simulink model "assignment_4"  (R2020b)
settings: Solver=VariableStepAuto  StartTime=0.0  StopTime=10.0  RelTol=1e-3
values from neighbouring files (symbols this model uses):
  b = 3.5077E-6    [dict1.sldd]
  J = 3.2284E-6    [dict1.sldd]
  K = 0.0274    [dict1.sldd]
  L = 2.75E-6    [dict1.sldd]
  R = 4.0    [dict1.sldd]
settings Model: Creator=Sudhanshu  LastModifiedBy=Sudhanshu

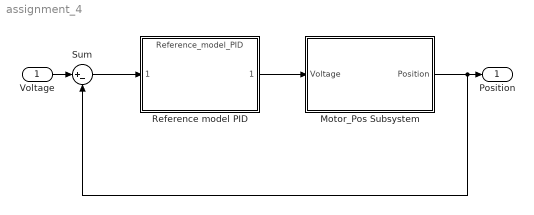
== system assignment_4 ==
  Voltage : Inport
  Motor_Pos Subsystem : Subsystem
  Reference model PID : ModelReference  ModelNameDialog=Reference_model_PID  SimulationMode=Normal  ModelReferenceVersion=1.4
  Sum : Sum  Inputs=|+-
  Position : Outport
  wires:
  Motor_Pos Subsystem/1(Position) -> Sum/2, Position/1
  Voltage/1 -> Sum/1
  Sum/1 -> Reference model PID/1
  Reference model PID/1 -> Motor_Pos Subsystem/1(Voltage)

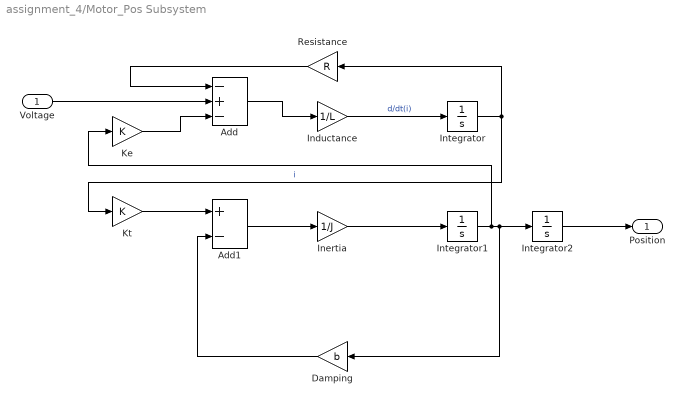
== system assignment_4/Motor_Pos Subsystem ==
  Voltage : Inport
  Add : Sum  Inputs=-+-
  Add1 : Sum  Inputs=+-
  Damping : Gain  Gain=b
  Inductance : Gain  Gain=1/L
  Inertia : Gain  Gain=1/J
  Integrator : Integrator
  Integrator1 : Integrator
  Integrator2 : Integrator
  Ke : Gain  Gain=K
  Kt : Gain  Gain=K
  Resistance : Gain  Gain=R
  Position : Outport
  wires:
  Inertia/1 -> Integrator1/1
  Kt/1 -> Add1/1
  Damping/1 -> Add1/2
  Ke/1 -> Add/3
  Add/1 -> Inductance/1
  Integrator1/1 -> Damping/1, Integrator2/1, Ke/1
  Add1/1 -> Inertia/1
  Resistance/1 -> Add/1
  Integrator/1 -> Resistance/1, Kt/1  "i"
  Inductance/1 -> Integrator/1  "d/dt(i)"
  Voltage/1 -> Add/2
  Integrator2/1 -> Position/1
